simulink model "dlb"  (R2017a)
settings: Solver=VariableStepAuto  StartTime=0.0  StopTime=10.0  RelTol=1e-3
values from neighbouring files (symbols this model uses):
  G = K'    [keshe6.m]
  K = acker(A,B,P)    [keshe6.m]    (also in keshe7.m = inv(Ph)*Vh)
  K1 = acker(A1,B1,ps)    [keshe1.m]    (also in keshe6.m = K(1:4))
  K2 = -K(5)    [keshe6.m]
settings Model: Creator=DELL  LastModifiedBy=adi
settings DataIOCC: ReturnWorkspaceOutputs=on
settings SFSimCC: SimUseLocalCustomCode=on
settings RTWCC: RTWUseLocalCustomCode=on

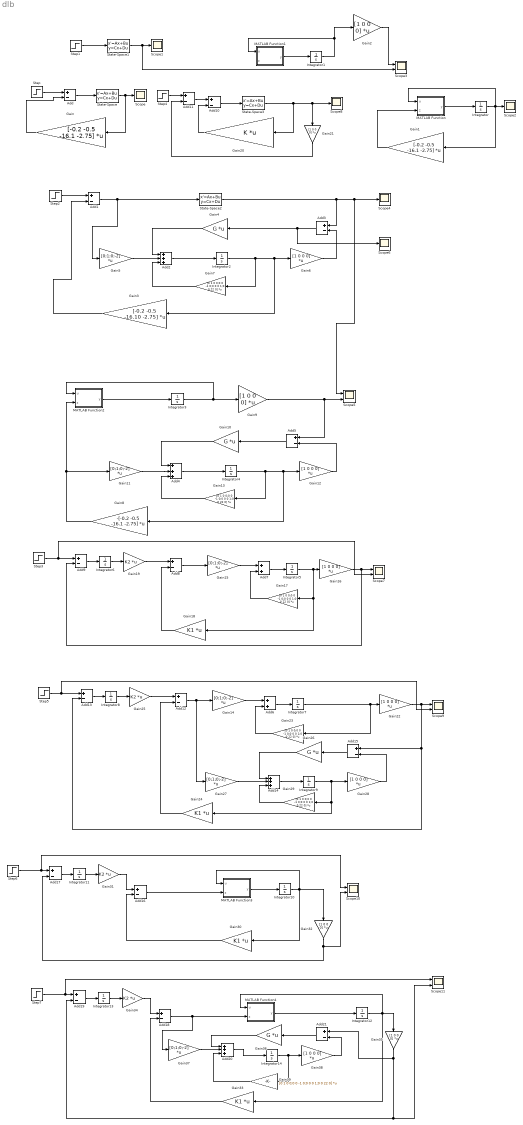
== system dlb ==
  Add{,1,3,5,8..13,15..19,21} (16 alike) : Sum  Inputs=+-
  Add{2,4,14,20} (4 alike) : Sum  Inputs=+++
  Add6 : Sum
  Add7 : Sum
  Gain : Gain  Gain=[-0.2 -0.5 -16.1 -2.75]  Multiplication=Matrix(K*u)
  Gain1 : Gain  Gain=[-0.2 -0.5 -16.1 -2.75]  Multiplication=Matrix(K*u)
  Gain{4,10,26,36} (4 alike) : Gain  Gain=G  Multiplication=Matrix(K*u)
  Gain{5,11,14..15,27,37} (6 alike) : Gain  Gain=[0;1;0;-2]  Multiplication=Matrix(K*u)
  Gain{2,6,9,12,16,21..22,28,32,35,38} (11 alike) : Gain  Gain=[1 0 0 0]  Multiplication=Matrix(K*u)
  Gain{7,13,17,23,29,39} (6 alike) : Gain  Gain=[0 1 0 0;0 0 -1 0;0 0 0 1;0 0 22 0]  Multiplication=Matrix(K*u)
  Gain{18,24,30,33} (4 alike) : Gain  Gain=K1  Multiplication=Matrix(K*u)
  Gain{19,25,31,34} (4 alike) : Gain  Gain=K2  Multiplication=Matrix(K*u)
  Gain20 : Gain  Gain=K  Multiplication=Matrix(K*u)
  Gain3 : Gain  Gain=[-0.2 -0.5 -16.10 -2.75]  Multiplication=Matrix(K*u)
  Gain8 : Gain  Gain=-[-0.2 -0.5 -16.1 -2.75]  Multiplication=Matrix(K*u)
  Integrator{,1..4} (5 alike) : Integrator  InitialCondition=[0.1 0.1 0.1 0.1]
  Integrator{5,7,9..10,12,14} (6 alike) : Integrator  InitialCondition=[0.1 0.1 0.1 0.1]*0
  Integrator{6,8,11,13} (4 alike) : Integrator
  MATLAB Function : MATLAB Function  TreatAsAtomicUnit=on
  MATLAB Function1 : MATLAB Function  TreatAsAtomicUnit=on
  MATLAB Function2 : MATLAB Function  TreatAsAtomicUnit=on
  MATLAB Function3 : MATLAB Function  TreatAsAtomicUnit=on
  MATLAB Function4 : MATLAB Function  TreatAsAtomicUnit=on
  Scope{,1..2,4,6,8} (6 alike) : Scope
  Scope{3,5,7,9..11} (6 alike) : Scope  NumInputPorts=2
  State-Space : StateSpace  A=[0 1 0 0;0 0 -1 0;0 0 0 1;0 0 22 0]  B=[0;1;0;-2]  C=[1 0 0 0;0 1 0 0;0 0 1 0;0 0 0 1]  D=[0;0;0;0]
  State-Space1 : StateSpace  A=[0 1 0 0;0 0 -1 0;0 0 0 1;0 0 22 0]  B=[0;1;0;-2]  C=[1 0 0 0]  D=0
  State-Space2 : StateSpace  A=[0 1 0 0;0 0 -1 0;0 0 0 1;0 0 22 0]  B=[0;1;0;-2]  C=[1 0 0 0]  D=0
  State-Space3 : StateSpace  A=[0 1 0 0;0 0 -1 0;0 0 0 1;0 0 22 0]  B=[0;1;0;-2]  C=[1 0 0 0;0 1 0 0;0 0 1 0;0 0 0 1]  D=[0;0;0;0]
  Step : Step  After=0  SampleTime=0
  Step{1,3..7} (6 alike) : Step  SampleTime=0
  Step2 : Step  After=0  SampleTime=0
  wires:
  Add/1 -> State-Space/1
  Step1/1 -> State-Space1/1
  State-Space1/1 -> Scope3/2, Scope1/1
  Gain/1 -> Add/2
  MATLAB Function1/1(y) -> Integrator1/1
  Integrator1/1 -> Gain2/1, MATLAB Function1/1(u)
  Gain2/1 -> Scope3/1
  Integrator/1 -> MATLAB Function/1(u), Gain1/1, Scope2/1
  MATLAB Function/1(y) -> Integrator/1
  Gain1/1 -> MATLAB Function/2(z)
  Add1/1 -> Gain5/1, State-Space2/1
  Gain3/1 -> Add1/2
  State-Space2/1 -> Add3/1, Scope5/1, Scope4/1
  Step2/1 -> Add1/1
  Integrator2/1 -> Gain7/1, Gain3/1, Gain6/1
  Add2/1 -> Integrator2/1
  Add3/1 -> Scope6/1, Gain4/1
  Gain6/1 -> Add3/2
  Gain7/1 -> Add2/3
  Gain5/1 -> Add2/2
  Gain4/1 -> Add2/1
  MATLAB Function2/1(y) -> Integrator3/1
  Gain8/1 -> Gain11/1, MATLAB Function2/2(z)
  Integrator3/1 -> MATLAB Function2/1(u), Gain9/1
  Add4/1 -> Integrator4/1
  Add5/1 -> Gain10/1
  Gain11/1 -> Add4/2
  Gain12/1 -> Add5/2
  Gain10/1 -> Add4/1
  Integrator4/1 -> Gain13/1, Gain8/1, Gain12/1
  Gain13/1 -> Add4/3
  Gain9/1 -> Add5/1, Scope5/2
  State-Space/1 -> Scope/1, Gain/1
  Gain15/1 -> Add7/1
  Add7/1 -> Integrator5/1
  Gain16/1 -> Add9/2, Scope7/1
  Integrator5/1 -> Gain18/1, Gain17/1, Gain16/1
  Gain17/1 -> Add7/2
  Add8/1 -> Gain15/1
  Gain18/1 -> Add8/2
  Gain19/1 -> Add8/1
  Integrator6/1 -> Gain19/1
  Add9/1 -> Integrator6/1
  Step3/1 -> Scope7/2, Add9/1
  Step4/1 -> Add11/1
  Add10/1 -> State-Space3/1
  Gain20/1 -> Add10/2
  Add11/1 -> Add10/1
  Step/1 -> Add/1
  State-Space3/1 -> Gain20/1, Gain21/1, Scope8/1
  Gain21/1 -> Add11/2
  Add6/1 -> Integrator7/1
  Gain22/1 -> Add15/1, Add13/2, Scope9/1
  Add12/1 -> Gain27/1, Gain14/1
  Integrator8/1 -> Gain25/1
  Gain23/1 -> Add6/2
  Add13/1 -> Integrator8/1
  Integrator7/1 -> Gain23/1, Gain22/1
  Step5/1 -> Scope9/2, Add13/1
  Gain14/1 -> Add6/1
  Gain25/1 -> Add12/1
  Gain24/1 -> Add12/2
  Gain27/1 -> Add14/2
  Gain28/1 -> Add15/2
  Add14/1 -> Integrator9/1
  Add15/1 -> Gain26/1
  Integrator9/1 -> Gain24/1, Gain29/1, Gain28/1
  Gain26/1 -> Add14/1
  Gain29/1 -> Add14/3
  Integrator10/1 -> MATLAB Function3/1(u), Gain30/1, Gain32/1
  Integrator11/1 -> Gain31/1
  Gain31/1 -> Add16/1
  Add17/1 -> Integrator11/1
  Add16/1 -> MATLAB Function3/2(z)
  Gain30/1 -> Add16/2
  Step6/1 -> Scope10/1, Add17/1
  Gain32/1 -> Scope10/2, Add17/2
  MATLAB Function3/1(y) -> Integrator10/1
  Step7/1 -> Scope11/1, Add19/1
  Add19/1 -> Integrator13/1
  Integrator13/1 -> Gain34/1
  Gain34/1 -> Add18/1
  Gain35/1 -> Scope11/2, Add19/2, Add21/1
  Integrator12/1 -> MATLAB Function4/1(u), Gain33/1, Gain35/1
  Add18/1 -> Gain37/1, MATLAB Function4/2(z)
  MATLAB Function4/1(y) -> Integrator12/1
  Gain33/1 -> Add18/2
  Add21/1 -> Gain36/1
  Add20/1 -> Integrator14/1
  Gain36/1 -> Add20/1
  Gain37/1 -> Add20/2
  Gain38/1 -> Add21/2
  Integrator14/1 -> Gain39/1, Gain38/1
  Gain39/1 -> Add20/3

== matlab function dlb/MATLAB Function1 ==
  data: u input; y output; z input
function y = fcn(u,z)
%#codegen
%x1=u(1);
%x2=u(2);
%x3=u(3);
%x4=u(4);
%dx1=x2;
%dx2=(-11sinx1+0.05sinx1cosx1x2)/(0.05cosx1*cosx1-0.55);
%dx3=x4;
%dx4=(0.05sinx1x2*x2-cosx1sinx1)/(1.1-0.1cosx1*cosx1);
%y=[dx1;dx2;dx3;dx4];

y = [u(2);
    (z*cos(u(1))-11*sin(u(1))+0.05*sin(u(1))*cos(u(1))*u(2)^2)/(0.05*cos(u(1))*cos(u(1))-0.55);
     u(4);
    (z+0.05*sin(u(1))*u(2)*u(2)-cos(u(1))*sin(u(1)))/(1.1-0.1*cos(u(1))*cos(u(1)))];

== matlab function dlb/MATLAB Function ==
  data: u input; y output; z input
function y = fcn(u,z)
%#codegen
%x1=u(1);
%x2=u(2);
%x3=u(3);   
%x4=u(4);
%dx1=x2;
%dx2=(-11sinx1+0.05sinx1cosx1x2)/(0.05cosx1*cosx1-0.55);
%dx3=x4;
%dx4=(0.05sinx1x2*x2-cosx1sinx1)/(1.1-0.1cosx1*cosx1);
%y=[dx1;dx2;dx3;dx4];

y = [u(2);
    (z*cos(u(1))-11*sin(u(1))+0.05*sin(u(1))*cos(u(1))*u(2)^2)/(0.05*cos(u(1))*cos(u(1))-0.55);
     u(4);
    (z+0.05*sin(u(1))*u(2)*u(2)-cos(u(1))*sin(u(1)))/(1.1-0.1*cos(u(1))*cos(u(1)))];

== matlab function dlb/MATLAB Function2 ==
  data: u input; y output; z input
function y = fcn(u,z)
%#codegen
%x1=u(1);
%x2=u(2);
%x3=u(3);
%x4=u(4);
%dx1=x2;
%dx2=(-11sinx1+0.05sinx1cosx1x2)/(0.05cosx1*cosx1-0.55);
%dx3=x4;
%dx4=(0.05sinx1x2*x2-cosx1sinx1)/(1.1-0.1cosx1*cosx1);
%y=[dx1;dx2;dx3;dx4];

y = [u(2);
    (z+0.05*sin(u(3))*u(4)*u(4)-cos(u(3))*sin(u(3)))/(1.1-0.1*cos(u(3))*cos(u(3)));
     u(4);
    (z*cos(u(3))-11*sin(u(3))+0.05*sin(u(3))*cos(u(3))*u(4)^2)/(0.05*cos(u(3))*cos(u(3))-0.55);];

== matlab function dlb/MATLAB Function3 ==
  data: u input; y output; z input
function y = fcn(u,z)
%#codegen
%x1=u(1);
%x2=u(2);
%x3=u(3);
%x4=u(4);
%dx1=x2;
%dx2=(-11sinx1+0.05sinx1cosx1x2)/(0.05cosx1*cosx1-0.55);
%dx3=x4;
%dx4=(0.05sinx1x2*x2-cosx1sinx1)/(1.1-0.1cosx1*cosx1);
%y=[dx1;dx2;dx3;dx4];

y = [u(2);
    (z+0.05*sin(u(3))*u(4)*u(4)-cos(u(3))*sin(u(3)))/(1.1-0.1*cos(u(3))*cos(u(3)));
     u(4);
    (z*cos(u(3))-11*sin(u(3))+0.05*sin(u(3))*cos(u(3))*u(4)^2)/(0.05*cos(u(3))*cos(u(3))-0.55);];

== matlab function dlb/MATLAB Function4 ==
  data: u input; y output; z input
function y = fcn(u,z)
%#codegen
%x1=u(1);
%x2=u(2);
%x3=u(3);
%x4=u(4);
%dx1=x2;
%dx2=(-11sinx1+0.05sinx1cosx1x2)/(0.05cosx1*cosx1-0.55);
%dx3=x4;
%dx4=(0.05sinx1x2*x2-cosx1sinx1)/(1.1-0.1cosx1*cosx1);
%y=[dx1;dx2;dx3;dx4];

y = [u(2);
    (z+0.05*sin(u(3))*u(4)*u(4)-cos(u(3))*sin(u(3)))/(1.1-0.1*cos(u(3))*cos(u(3)));
     u(4);
    (z*cos(u(3))-11*sin(u(3))+0.05*sin(u(3))*cos(u(3))*u(4)^2)/(0.05*cos(u(3))*cos(u(3))-0.55);];
